simulink model "attitude_controllerV6"  (R2025a)
settings: Solver=FixedStepDiscrete  StartTime=0.0  StopTime=40  FixedStep=1e-4  RelTol=1e-6
undefined symbols (not defined in the file or in its folder): DiscIntNeverNeededParam
libraries: simulink x18, cstblocks x14, slpidlib x6, aerolibutil x2, rllib x1
(part 1 of 2)
settings Model: Creator=Rewse  LastModifiedBy=Rewse
settings SolverCC: ZeroCrossAlgorithm=Adaptive
settings DebuggingCC: IgnoredZcDiagnostic=none

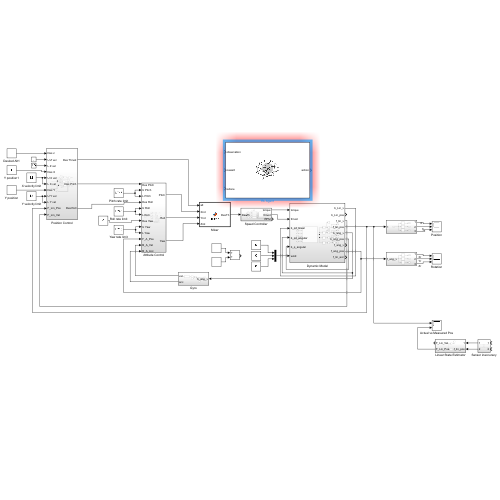
[thumbnail: Simulink's stored preview of the top-level diagram]
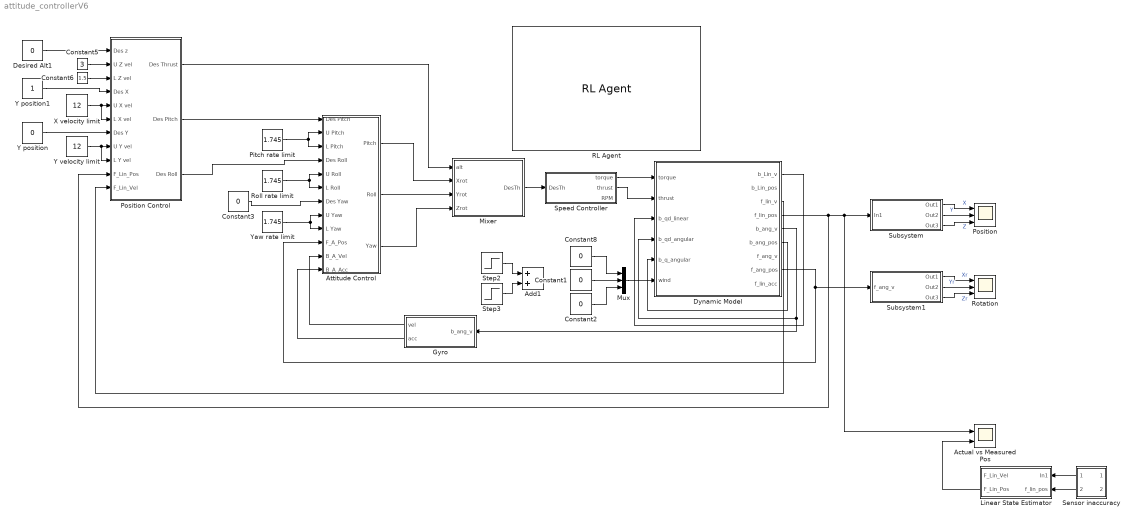
== system attitude_controllerV6 ==
  Actual vs Measured Pos : Scope  NumInputPorts=2
      settings: ActiveDisplayYMinimum=-0.72419600366773873  ActiveDisplayYMaximum=1.3775619520636175  DataLoggingVariableName=ScopeData20
  Add1 : Sum
  Attitude Control : Subsystem
  Constant{1..3,8} (4 alike) : Constant  Value=0
  Constant5 : Constant  Value=3
  Constant6 : Constant  Value=1.5
  Desired Alt1 : Constant  Value=0
  Dynamic Model : Subsystem
  Gyro : Subsystem
  Linear State Estimator : Subsystem
  Mixer : MATLAB Function  TreatAsAtomicUnit=on
  Mux : Mux  Inputs=3
  Pitch rate limit : Constant  Value=1.745
  Position : Scope  NumInputPorts=3
      settings: ActiveDisplayYMinimum=-0.995943473561637  ActiveDisplayYMaximum=3.6382297992423651
  Position Control : Subsystem
  RL Agent : rllib/RL Agent  Agent=agentObj  ExternalActionAsInput=off  ProvideLastAction=off  ProvideCumRwd=off  TreatAsDirectFeedthrough=on  UseStrictObservationDataTypes=off
  Roll rate limit : Constant  Value=1.745
  Rotation : Scope  NumInputPorts=3
      settings: ActiveDisplayYMinimum=-0.95912404587525768  ActiveDisplayYMaximum=0.95521723280052528
  Sensor inaccuracy : Subsystem
  Speed Controller : Subsystem
  Step2 : Step  After=15  SampleTime=2
  Step3 : Step  Time=8  After=-15  SampleTime=3
  Subsystem : Subsystem
  Subsystem1 : Subsystem
  X velocity limit : Constant  Value=12
  Y position : Constant  Value=0
  Y position1 : Constant
  Y velocity limit : Constant  Value=12
  Yaw rate limit : Constant  Value=1.745
  wires:
  Subsystem/1(Out1) -> Position/1  "X"
  Subsystem/2(Out2) -> Position/2  "Y"
  Subsystem/3(Out3) -> Position/3  "Z"
  Subsystem1/1(Out1) -> Rotation/1  "Xr"
  Subsystem1/2(Out2) -> Rotation/2  "Yr"
  Subsystem1/3(Out3) -> Rotation/3  "Zr"
  Dynamic Model/6(b_ang_pos) -> Dynamic Model/5(b_q_angular)
  Dynamic Model/1(b_Lin_v) -> Dynamic Model/3(b_qd_linear)
  Mixer/1(DesTh) -> Speed Controller/1(DesTh)
  Dynamic Model/5(b_ang_v) -> Dynamic Model/4(b_qd_angular), Gyro/1(b_ang_v)
  Attitude Control/1(Pitch) -> Mixer/2(Xrot)
  Attitude Control/2(Roll) -> Mixer/3(Yrot)
  Pitch rate limit/1 -> Attitude Control/3(L Pitch), Attitude Control/2(U Pitch)
  Roll rate limit/1 -> Attitude Control/6(L Roll), Attitude Control/5(U Roll)
  Yaw rate limit/1 -> Attitude Control/9(L Yaw), Attitude Control/8(U Yaw)
  Constant3/1 -> Attitude Control/7(Des Yaw)
  Mux/1 -> Dynamic Model/6(wind)
  Speed Controller/2(thrust) -> Dynamic Model/2(thrust)
  Speed Controller/1(torque) -> Dynamic Model/1(torque)
  Constant5/1 -> Position Control/2(U Z vel)
  Desired Alt1/1 -> Position Control/1(Des z)
  X velocity limit/1 -> Position Control/6(L X vel), Position Control/5(U X vel)
  Y velocity limit/1 -> Position Control/9(L Y vel), Position Control/8(U Y vel)
  Position Control/1(Des Thrust) -> Mixer/1(alt)
  Constant6/1 -> Position Control/3(L Z vel)
  Y position/1 -> Position Control/7(Des Y)
  Attitude Control/3(Yaw) -> Mixer/4(Zrot)
  Gyro/1(vel) -> Attitude Control/11(B_A_Vel)
  Gyro/2(acc) -> Attitude Control/12(B_A_Acc)
  Dynamic Model/8(f_ang_pos) -> Attitude Control/10(F_A_Pos), Subsystem1/1(f_ang_v)
  Y position1/1 -> Position Control/4(Des X)
  Constant2/1 -> Mux/3
  Constant8/1 -> Mux/1
  Step2/1 -> Add1/1
  Step3/1 -> Add1/2
  Sensor inaccuracy/2(Out2) -> Linear State Estimator/2(f_lin_pos)
  Sensor inaccuracy/1(Out1) -> Linear State Estimator/1(In1)
  Dynamic Model/3(f_lin_v) -> Position Control/11(F_Lin_Vel)
  Constant1/1 -> Mux/2
  Linear State Estimator/2(F_Lin_Pos) -> Actual vs Measured Pos/2
  Position Control/3(Des Roll) -> Attitude Control/4(Des Roll)
  Position Control/2(Des Pitch) -> Attitude Control/1(Des Pitch)
  Dynamic Model/4(f_lin_pos) -> Position Control/10(F_Lin_Pos), Actual vs Measured Pos/1, Subsystem/1(In1)

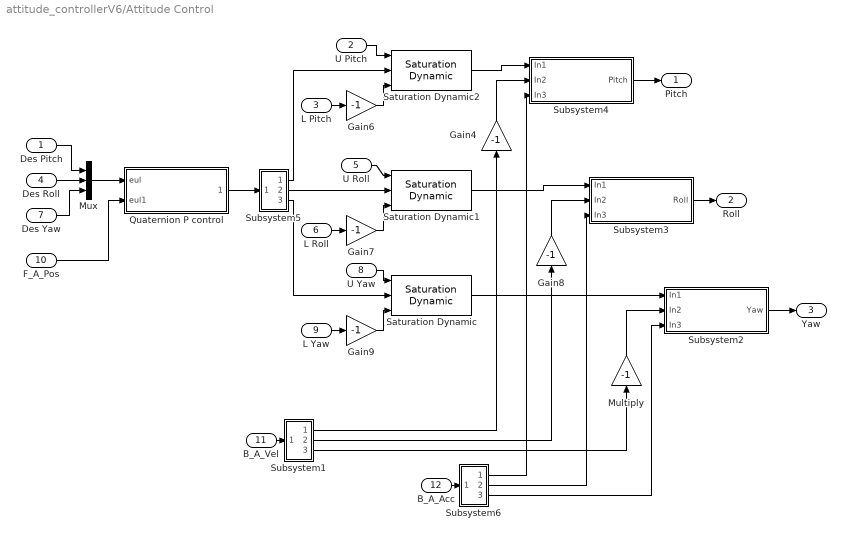
== system attitude_controllerV6/Attitude Control ==
  Des Pitch : Inport
  U Pitch : Inport  Port=2
  L Pitch : Inport  Port=3
  Des Roll : Inport  Port=4
  U Roll : Inport  Port=5
  L Roll : Inport  Port=6
  Des Yaw : Inport  Port=7
  U Yaw : Inport  Port=8
  L Yaw : Inport  Port=9
  F_A_Pos : Inport  Port=10
  B_A_Vel : Inport  Port=11
  B_A_Acc : Inport  Port=12
  Gain{4,6..9} (5 alike) : Gain  Gain=-1
  Multiply : Gain  Gain=-1
  Mux : Mux  Inputs=3
  Quaternion P control : Subsystem
  Saturation Dynamic : simulink/Discontinuities/Saturation Dynamic  OutMin=[]  OutMax=[]  OutDataTypeStr=Inherit: Same as second input  OutDataType=fixdt(1, 16)  OutScaling=2^-10  DoSatur=off
  Saturation Dynamic1 : simulink/Discontinuities/Saturation Dynamic  OutMin=[]  OutMax=[]  OutDataTypeStr=Inherit: Same as second input  OutDataType=fixdt(1, 16)  OutScaling=2^-10  DoSatur=off
  Saturation Dynamic2 : simulink/Discontinuities/Saturation Dynamic  OutMin=[]  OutMax=[]  OutDataTypeStr=Inherit: Same as second input  OutDataType=fixdt(1, 16)  OutScaling=2^-10  DoSatur=off
  Subsystem1 : Subsystem
  Subsystem2 : Subsystem
  Subsystem3 : Subsystem
  Subsystem4 : Subsystem
  Subsystem5 : Subsystem
  Subsystem6 : Subsystem
  Pitch : Outport
  Roll : Outport  Port=2
  Yaw : Outport  Port=3
  wires:
  Gain9/1 -> Saturation Dynamic/3
  Gain6/1 -> Saturation Dynamic2/3
  Gain7/1 -> Saturation Dynamic1/3
  B_A_Vel/1 -> Subsystem1/1("  ")
  U Roll/1 -> Saturation Dynamic1/1
  L Pitch/1 -> Gain6/1
  U Pitch/1 -> Saturation Dynamic2/1
  Subsystem1/1(Out1) -> Gain4/1
  Subsystem1/2(Out2) -> Gain8/1
  Subsystem1/3(Out3) -> Multiply/1
  Saturation Dynamic/1 -> Subsystem2/1(In1)
  Gain8/1 -> Subsystem3/2(In2)
  Subsystem2/1(Yaw) -> Yaw/1
  Multiply/1 -> Subsystem2/2(In2)
  Gain4/1 -> Subsystem4/2(In2)
  Subsystem4/1(Pitch) -> Pitch/1
  Saturation Dynamic1/1 -> Subsystem3/1(In1)
  Subsystem3/1(Roll) -> Roll/1
  L Yaw/1 -> Gain9/1
  Des Pitch/1 -> Mux/1
  Des Roll/1 -> Mux/2
  Des Yaw/1 -> Mux/3
  U Yaw/1 -> Saturation Dynamic/1
  Subsystem5/3(Out3) -> Saturation Dynamic/2
  Subsystem5/2(Out2) -> Saturation Dynamic1/2
  Subsystem5/1(Out1) -> Saturation Dynamic2/2
  Mux/1 -> Quaternion P control/1(eul)
  F_A_Pos/1 -> Quaternion P control/2(eul1)
  Quaternion P control/1("  ") -> Subsystem5/1("  ")
  L Roll/1 -> Gain7/1
  Saturation Dynamic2/1 -> Subsystem4/1(In1)
  B_A_Acc/1 -> Subsystem6/1("  ")
  Subsystem6/1(Out1) -> Subsystem4/3(In3)
  Subsystem6/2(Out2) -> Subsystem3/3(In3)
  Subsystem6/3(Out3) -> Subsystem2/3(In3)

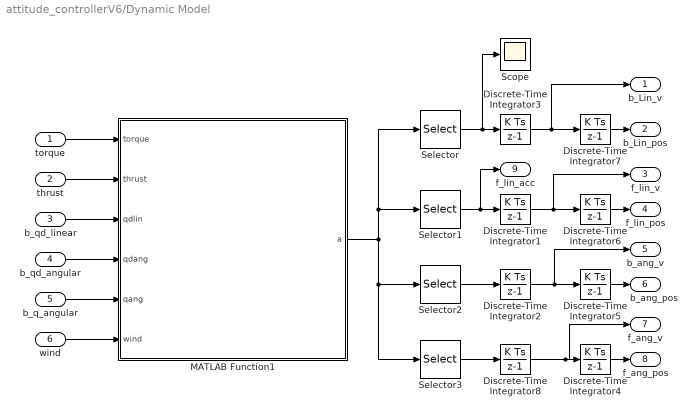
== system attitude_controllerV6/Dynamic Model ==
  torque : Inport
  thrust : Inport  Port=2
  b_qd_linear : Inport  Port=3
  b_qd_angular : Inport  Port=4
  b_q_angular : Inport  Port=5
  wind : Inport  Port=6
  Discrete-Time Integrator{1..8} (8 alike) : DiscreteIntegrator  SampleTime=-1  ICPrevOutput=DiscIntNeverNeededParam  ICPrevScaledInput=DiscIntNeverNeededParam
  MATLAB Function1 : MATLAB Function  TreatAsAtomicUnit=on
  Scope : Scope
      settings: ActiveDisplayYMinimum=-1  ActiveDisplayYMaximum=1  DataLoggingVariableName=ScopeData3
  Selector : Selector  InputPortWidth=12  IndexOptions=Index vector (dialog)  Indices=[1 2 3]  OutputSizes=1
  Selector1 : Selector  InputPortWidth=12  IndexOptions=Index vector (dialog)  Indices=[4 5 6]  OutputSizes=1
  Selector2 : Selector  InputPortWidth=12  IndexOptions=Index vector (dialog)  Indices=[7 8 9]  OutputSizes=1
  Selector3 : Selector  InputPortWidth=12  IndexOptions=Index vector (dialog)  Indices=[10 11 12]  OutputSizes=1
  b_Lin_v : Outport
  b_Lin_pos : Outport  Port=2
  f_lin_v : Outport  Port=3
  f_lin_pos : Outport  Port=4
  b_ang_v : Outport  Port=5
  b_ang_pos : Outport  Port=6
  f_ang_v : Outport  Port=7
  f_ang_pos : Outport  Port=8
  f_lin_acc : Outport  Port=9
  wires:
  torque/1 -> MATLAB Function1/1(torque)
  thrust/1 -> MATLAB Function1/2(thrust)
  b_qd_linear/1 -> MATLAB Function1/3(qdlin)
  b_qd_angular/1 -> MATLAB Function1/4(qdang)
  b_q_angular/1 -> MATLAB Function1/5(qang)
  wind/1 -> MATLAB Function1/6(wind)
  MATLAB Function1/1(a) -> Selector1/1, Selector/1, Selector3/1, Selector2/1
  Selector/1 -> Scope/1, Discrete-Time Integrator3/1
  Selector1/1 -> f_lin_acc/1, Discrete-Time Integrator1/1
  Selector2/1 -> Discrete-Time Integrator2/1
  Selector3/1 -> Discrete-Time Integrator8/1
  Discrete-Time Integrator3/1 -> Discrete-Time Integrator7/1, b_Lin_v/1
  Discrete-Time Integrator7/1 -> b_Lin_pos/1
  Discrete-Time Integrator2/1 -> b_ang_v/1, Discrete-Time Integrator5/1
  Discrete-Time Integrator1/1 -> Discrete-Time Integrator6/1, f_lin_v/1
  Discrete-Time Integrator8/1 -> f_ang_v/1, Discrete-Time Integrator4/1
  Discrete-Time Integrator4/1 -> f_ang_pos/1
  Discrete-Time Integrator5/1 -> b_ang_pos/1
  Discrete-Time Integrator6/1 -> f_lin_pos/1

== system attitude_controllerV6/Gyro ==
  b_ang_v : Inport
  Constant1 : Constant  Value=40
  Constant7 : Constant  Value=40
  Discrete Derivative : simulink/Discrete/Discrete Derivative  gainval=1.0  ICPrevScaledInput=0.0  OutMin=[]  OutMax=[]  OutDataType=fixdt(1, 16)  OutScaling=2^-10  DoSatur=off
  Discrete Varying Lowpass : cstblocks/Linear Parameter Varying/Discrete Varying Lowpass  N=2  w0=0  Ts=1e-3
  Discrete Varying Lowpass1 : cstblocks/Linear Parameter Varying/Discrete Varying Lowpass  N=2  w0=0  Ts=1e-3
  Quantizer : Quantizer  QuantizationInterval=0.00026179939
  noise : Subsystem
  vel : Outport
  acc : Outport  Port=2
  wires:
  Constant1/1 -> Discrete Varying Lowpass1/2
  Quantizer/1 -> Discrete Varying Lowpass/1
  Discrete Derivative/1 -> Discrete Varying Lowpass1/1
  Constant7/1 -> Discrete Varying Lowpass/2
  Discrete Varying Lowpass/1 -> vel/1, Discrete Derivative/1
  b_ang_v/1 -> noise/1(In1)
  noise/1(Out1) -> Quantizer/1
  Discrete Varying Lowpass1/1 -> acc/1

== system attitude_controllerV6/Linear State Estimator ==
  In1 : Inport
  f_lin_pos : Inport  Port=2
  Complimentary filter : Subsystem
  Constant7 : Constant  Value=10
  Discrete Varying Lowpass1 : cstblocks/Linear Parameter Varying/Discrete Varying Lowpass  N=2  w0=0  Ts=1e-3
  Scope : Scope
      settings: ActiveDisplayYMinimum=-0.34461683334154741  ActiveDisplayYMaximum=0.3611283671784512  DataLoggingVariableName=ScopeData17
  F_Lin_Vel : Outport
  F_Lin_Pos : Outport  Port=2
  wires:
  In1/1 -> Discrete Varying Lowpass1/1, Complimentary filter/1(In1)
  f_lin_pos/1 -> Complimentary filter/2(f_lin_pos)
  Complimentary filter/1(F_Lin_Pos) -> F_Lin_Pos/1
  Discrete Varying Lowpass1/1 -> Scope/1, F_Lin_Vel/1
  Constant7/1 -> Discrete Varying Lowpass1/2

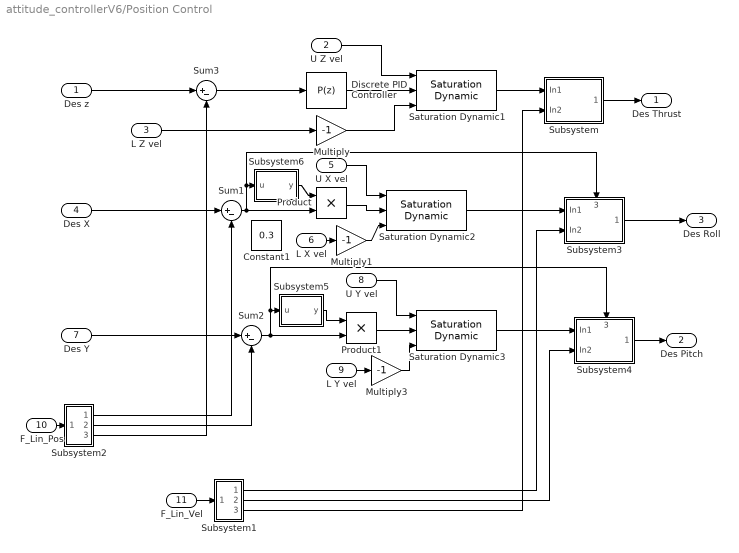
== system attitude_controllerV6/Position Control ==
  Des z : Inport
  U Z vel : Inport  Port=2
  L Z vel : Inport  Port=3
  Des X : Inport  Port=4
  U X vel : Inport  Port=5
  L X vel : Inport  Port=6
  Des Y : Inport  Port=7
  U Y vel : Inport  Port=8
  L Y vel : Inport  Port=9
  F_Lin_Pos : Inport  Port=10
  F_Lin_Vel : Inport  Port=11
  Constant1 : Constant  Value=0.3
  Discrete PID Controller : slpidlib/PID Controller  Controller=P  Form=Parallel  TimeDomain=Discrete-time  UseExternalTs=off  SampleTime=-1  IntegratorMethod=Forward Euler  FilterMethod=Forward Euler  ControllerParametersSource=internal  P=4  I=0.2  UseKiTs=off  D=1  UseExternalDerivativeSource=off  N=100  UseFilter=on  TunerSelectOption=Transfer Function Based (PID Tuner App)  InitialConditionSource=internal  InitialConditionForIntegrator=0  InitialConditionForFilter=0  DifferentiatorICPrevScaledInput=0  ExternalReset=none  TrackingMode=off  Kt=1  LimitOutput=off  SatLimitsSource=internal  UpperSaturationLimit=inf  LowerSaturationLimit=-inf  LinearizeAsGain=off  AntiWindupMode=none  Kb=1  LimitIntegrator=off  UpperIntegratorSaturationLimit=inf  LowerIntegratorSaturationLimit=-inf  POutMin=[]  POutMax=[]  IOutMin=[]  IOutMax=[]  DOutMin=[]  DOutMax=[]  NOutMin=[]  NOutMax=[]  SumOutMin=[]  SumOutMax=[]  SaturationOutMin=[]  SaturationOutMax=[]  PParamMin=[]  PParamMax=[]  IParamMin=[]  IParamMax=[]  DParamMin=[]  DParamMax=[]  NParamMin=[]  NParamMax=[]  KbParamMin=[]  KbParamMax=[]  KtParamMin=[]  KtParamMax=[]  KbOutMin=[]  KbOutMax=[]  KtOutMin=[]  KtOutMax=[]  IntegratorOutMin=[]  IntegratorOutMax=[]  FilterOutMin=[]  FilterOutMax=[]  SumI1OutMin=[]  SumI1OutMax=[]  SumI2OutMin=[]  SumI2OutMax=[]  SumI3OutMin=[]  SumI3OutMax=[]  SumI4OutMin=[]  SumI4OutMax=[]  SumDOutMin=[]  SumDOutMax=[]  DifferentiatorOutMin=[]  DifferentiatorOutMax=[]  FilterDiffOutCoefMin=[]  FilterDiffOutCoefMax=[]  ReciprocalOutMin=[]  ReciprocalOutMax=[]  SumDenOutMin=[]  SumDenOutMax=[]  SumNumOutMin=[]  SumNumOutMax=[]  DivideOutMin=[]  DivideOutMax=[]  UdiffTsProdOutMin=[]  UdiffTsProdOutMax=[]  NTsProdOutMin=[]  NTsProdOutMax=[]  UintegralTsProdOutMin=[]  UintegralTsProdOutMax=[]  UngainTsProdOutMin=[]  UngainTsProdOutMax=[]  ClampingZeroOutDataTypeStr=Inherit: Inherit via back propagation  ClampingZeroOutMin=[]  ClampingZeroOutMax=[]  FilterDenConstantOutDataTypeStr=Inherit: Inherit via back propagation  FilterDenConstantOutMin=[]  FilterDenConstantOutMax=[]  PCopyOutDataTypeStr=Inherit: Inherit via back propagation  PCopyOutMin=[]  PCopyOutMax=[]  NCopyOutDataTypeStr=Inherit: Inherit via back propagation  NCopyOutMin=[]  NCopyOutMax=[]  IntegratorContinuousStateAttributes=''  IntegratorStateMustResolveToSignalObject=off  IntegratorRTWStateStorageClass=Auto  FilterContinuousStateAttributes=''  FilterStateMustResolveToSignalObject=off  FilterRTWStateStorageClass=Auto  ParallelPVariant=InternalParameters  IdealPVariant=Disabled  IVariant=Disabled  DVariant=Disabled  IntegratorVariant=Disabled  SatVariant=Disabled  AWVariant=Disabled  PCopyVariant=Disabled  TRVariant=Disabled  FdbkBlocksVariant=Forward  IdealPFdbkVariant=Disabled  SatFdbkVariant=Disabled  DerivativeFilterVariant=Disabled  NVariant=Disabled  NCopyVariant=Disabled_SignalSpec  FilterICVariant=Disabled  IntegratorICVariant=Disabled  ExternalResetVariant=Disabled  TRSumVariant=Passthrough  SumFdbkVariant=Disabled  SumVariant=Passthrough_P  TsampFilterVariant=InternalTs  TsampNgainVariant=Passthrough  TsampIntegralVariant=Disabled_SignalSpec  ExternalSaturationOutDataTypeStr=Inherit: Same as second input  DerivativeSourceVariant=Disabled  PreIntVariant=InternalPreInt
      settings: LibrarySourceBlock=simulink/Discrete/Discrete PID Controller
  Multiply : Gain  Gain=-1
  Multiply1 : Gain  Gain=-1
  Multiply3 : Gain  Gain=-1
  Product : Product
  Product1 : Product
  Saturation Dynamic1 : simulink/Discontinuities/Saturation Dynamic  OutMin=[]  OutMax=[]  OutDataTypeStr=Inherit: Same as second input  OutDataType=fixdt(1, 16)  OutScaling=2^-10  DoSatur=off
  Saturation Dynamic2 : simulink/Discontinuities/Saturation Dynamic  OutMin=[]  OutMax=[]  OutDataTypeStr=Inherit: Same as second input  OutDataType=fixdt(1, 16)  OutScaling=2^-10  DoSatur=off
  Saturation Dynamic3 : simulink/Discontinuities/Saturation Dynamic  OutMin=[]  OutMax=[]  OutDataTypeStr=Inherit: Same as second input  OutDataType=fixdt(1, 16)  OutScaling=2^-10  DoSatur=off
  Subsystem : Subsystem
  Subsystem1 : Subsystem
  Subsystem2 : Subsystem
  Subsystem3 : Subsystem
      settings: PortSchema="{\"entries\":[{\"content\":{\"sides\":[{\"content\":{\"connectorIds\":[\"In1\",\"In2\"]},\"type\":\"ConnectorPlacement.EquallySpacedRectSide\",\"uuid\":\"8f94e582-882b-486f-b435-c6f08064346b\"},{\"content\":{\"connectorIds\":[\"Out1\"],\"side\":\"RIGHT\"},\"type\":\"ConnectorPlacement.EquallySpacedRectSide\",\"uuid\":\"472883df-7159-496e-9a5d-2a26c086a4a5\"},{\"content\":{\"connectorIds\":[\"In3\"],\"side\":\"TOP\"},\"type\":\"ConnectorPlacement.EquallySpacedRectSide\",\"uuid\":\"9ed532c8-9328-48c4-bd89-739726c76bc0\"}]},\"type\":\"ConnectorPlacement.EquallySpacedConnector\",\"uuid\":\"e990e484-f5ed-4898-afa7-038328da9bdf\"}],\"packageUris\":[\"http://schema.mathworks.com/mf0/Connector/R2020b\"],\"version\":\"1.0\"}"
  Subsystem4 : Subsystem
      settings: PortSchema="{\"entries\":[{\"content\":{\"sides\":[{\"content\":{\"connectorIds\":[\"In1\",\"In2\"]},\"type\":\"ConnectorPlacement.EquallySpacedRectSide\",\"uuid\":\"8f94e582-882b-486f-b435-c6f08064346b\"},{\"content\":{\"connectorIds\":[\"Out1\"],\"side\":\"RIGHT\"},\"type\":\"ConnectorPlacement.EquallySpacedRectSide\",\"uuid\":\"472883df-7159-496e-9a5d-2a26c086a4a5\"},{\"content\":{\"connectorIds\":[\"In3\"],\"side\":\"TOP\"},\"type\":\"ConnectorPlacement.EquallySpacedRectSide\",\"uuid\":\"9ed532c8-9328-48c4-bd89-739726c76bc0\"}]},\"type\":\"ConnectorPlacement.EquallySpacedConnector\",\"uuid\":\"e990e484-f5ed-4898-afa7-038328da9bdf\"}],\"packageUris\":[\"http://schema.mathworks.com/mf0/Connector/R2020b\"],\"version\":\"1.0\"}"
  Subsystem5 : Subsystem
  Subsystem6 : Subsystem
  Sum1 : Sum  Inputs=|+-
  Sum2 : Sum  Inputs=|+-
  Sum3 : Sum  Inputs=|+-
  Des Thrust : Outport
  Des Pitch : Outport  Port=2
  Des Roll : Outport  Port=3
  wires:
  Sum3/1 -> Discrete PID Controller/1
  Multiply/1 -> Saturation Dynamic1/3
  Des z/1 -> Sum3/1
  Discrete PID Controller/1 -> Saturation Dynamic1/2
  L Z vel/1 -> Multiply/1
  U Z vel/1 -> Saturation Dynamic1/1
  Saturation Dynamic1/1 -> Subsystem/1(In1)
  F_Lin_Vel/1 -> Subsystem1/1("  ")
  F_Lin_Pos/1 -> Subsystem2/1("  ")
  Subsystem2/3(Out3) -> Sum3/2
  Subsystem1/3(Out3) -> Subsystem/2(In2)
  Subsystem/1(Des Thrust) -> Des Thrust/1
  Des X/1 -> Sum1/1
  Sum1/1 -> Subsystem3/3(3), Subsystem6/1(u), Product/2
  Product/1 -> Saturation Dynamic2/2
  U X vel/1 -> Saturation Dynamic2/1
  Multiply1/1 -> Saturation Dynamic2/3
  L X vel/1 -> Multiply1/1
  Saturation Dynamic2/1 -> Subsystem3/1(In1)
  L Y vel/1 -> Multiply3/1
  Multiply3/1 -> Saturation Dynamic3/3
  Sum2/1 -> Subsystem5/1(u), Subsystem4/3(3), Product1/2
  Product1/1 -> Saturation Dynamic3/2
  Saturation Dynamic3/1 -> Subsystem4/1(In1)
  Subsystem4/1(Des Pitch) -> Des Pitch/1
  Des Y/1 -> Sum2/1
  U Y vel/1 -> Saturation Dynamic3/1
  Subsystem1/2(Out2) -> Subsystem4/2(In2)
  Subsystem1/1(Out1) -> Subsystem3/2(In2)
  Subsystem2/2(Out1) -> Sum2/2
  Subsystem2/1(Out2) -> Sum1/2
  Subsystem3/1(Des Roll) -> Des Roll/1
  Subsystem6/1(y) -> Product/1
  Subsystem5/1(y) -> Product1/1

== system attitude_controllerV6/Sensor inaccuracy ==
  In1 : Inport
  In2 : Inport  Port=2
  Quantizer : Quantizer  QuantizationInterval=0.01
  Quantizer1 : Quantizer  QuantizationInterval=1
  Out1 : Outport
  Out2 : Outport  Port=2
  wires:
  In1/1 -> Quantizer/1
  In2/1 -> Quantizer1/1
  Quantizer1/1 -> Out2/1
  Quantizer/1 -> Out1/1

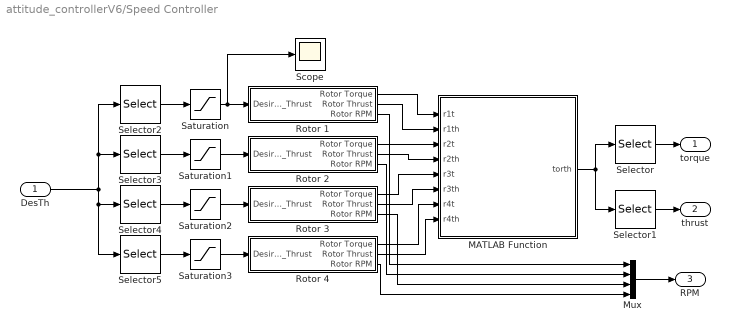
== system attitude_controllerV6/Speed Controller ==
  DesTh : Inport
  MATLAB Function : MATLAB Function  TreatAsAtomicUnit=on
  Mux : Mux
  Rotor 1 : Subsystem
  Rotor 2 : Subsystem
  Rotor 3 : Subsystem
  Rotor 4 : Subsystem
  Saturation{,1..3} (4 alike) : Saturate  UpperLimit=8.96325  LowerLimit=0
  Scope : Scope
      settings: ActiveDisplayYMinimum=-0.6431468749999999  ActiveDisplayYMaximum=5.788321875  DataLoggingVariableName=ScopeData6
  Selector : Selector  InputPortWidth=4  IndexOptions=Index vector (dialog)  Indices=[1 2 3]  OutputSizes=1
  Selector1 : Selector  InputPortWidth=4  IndexOptions=Index vector (dialog)  Indices=[4]  OutputSizes=1
  Selector2 : Selector  InputPortWidth=4  IndexOptions=Index vector (dialog)  Indices=[1]  OutputSizes=1
  Selector3 : Selector  InputPortWidth=4  IndexOptions=Index vector (dialog)  Indices=[2]  OutputSizes=1
  Selector4 : Selector  InputPortWidth=4  IndexOptions=Index vector (dialog)  Indices=[3]  OutputSizes=1
  Selector5 : Selector  InputPortWidth=4  IndexOptions=Index vector (dialog)  Indices=[4]  OutputSizes=1
  torque : Outport
  thrust : Outport  Port=2
  RPM : Outport  Port=3
  wires:
  DesTh/1 -> Selector5/1, Selector4/1, Selector3/1, Selector2/1
  Selector5/1 -> Saturation3/1
  Rotor 1/1(Rotor Torque) -> MATLAB Function/1(r1t)
  Selector2/1 -> Saturation/1
  Rotor 3/1(Rotor Torque) -> MATLAB Function/5(r3t)
  Selector3/1 -> Saturation1/1
  Rotor 1/2(Rotor Thrust) -> MATLAB Function/2(r1th)
  Selector4/1 -> Saturation2/1
  Rotor 2/1(Rotor Torque) -> MATLAB Function/3(r2t)
  MATLAB Function/1(torth) -> Selector/1, Selector1/1
  Selector1/1 -> thrust/1
  Selector/1 -> torque/1
  Saturation/1 -> Scope/1, Rotor 1/1(Desired_Thrust)
  Saturation1/1 -> Rotor 2/1(Desired_Thrust)
  Saturation2/1 -> Rotor 3/1(Desired_Thrust)
  Saturation3/1 -> Rotor 4/1(Desired_Thrust)
  Rotor 2/2(Rotor Thrust) -> MATLAB Function/4(r2th)
  Rotor 3/2(Rotor Thrust) -> MATLAB Function/6(r3th)
  Rotor 4/1(Rotor Torque) -> MATLAB Function/7(r4t)
  Rotor 4/2(Rotor Thrust) -> MATLAB Function/8(r4th)
  Rotor 1/3(Rotor RPM) -> Mux/1
  Rotor 2/3(Rotor RPM) -> Mux/2
  Rotor 3/3(Rotor RPM) -> Mux/3
  Rotor 4/3(Rotor RPM) -> Mux/4
  Mux/1 -> RPM/1

== system attitude_controllerV6/Subsystem ==
  In1 : Inport
  Selector1 : Selector  InputPortWidth=3  IndexOptions=Index vector (dialog)  Indices=[2]  OutputSizes=1
  Selector10 : Selector  InputPortWidth=3  IndexOptions=Index vector (dialog)  Indices=[1]  OutputSizes=1
  Selector2 : Selector  InputPortWidth=3  IndexOptions=Index vector (dialog)  Indices=[3]  OutputSizes=1
  Out1 : Outport
  Out2 : Outport  Port=2
  Out3 : Outport  Port=3
  wires:
  Selector10/1 -> Out1/1  "Xpos"
  Selector1/1 -> Out2/1  "Ypos"
  In1/1 -> Selector2/1, Selector10/1, Selector1/1
  Selector2/1 -> Out3/1  "Zpos"

== system attitude_controllerV6/Subsystem1 ==
  f_ang_v : Inport
  Selector1 : Selector  InputPortWidth=3  IndexOptions=Index vector (dialog)  Indices=[2]  OutputSizes=1
  Selector10 : Selector  InputPortWidth=3  IndexOptions=Index vector (dialog)  Indices=[1]  OutputSizes=1
  Selector2 : Selector  InputPortWidth=3  IndexOptions=Index vector (dialog)  Indices=[3]  OutputSizes=1
  Out1 : Outport
  Out2 : Outport  Port=2
  Out3 : Outport  Port=3
  wires:
  Selector10/1 -> Out1/1  "Xpos"
  Selector1/1 -> Out2/1  "Ypos"
  f_ang_v/1 -> Selector2/1, Selector10/1, Selector1/1
  Selector2/1 -> Out3/1  "Zpos"

== system attitude_controllerV6/Attitude Control/Quaternion P control ==
  eul : Inport
  eul1 : Inport  Port=2
  Discrete PID Controller1 : slpidlib/PID Controller  Controller=P  Form=Parallel  TimeDomain=Discrete-time  UseExternalTs=off  SampleTime=-1  IntegratorMethod=Forward Euler  FilterMethod=Forward Euler  ControllerParametersSource=internal  P=2  I=1  UseKiTs=off  D=0  UseExternalDerivativeSource=off  N=100  UseFilter=on  TunerSelectOption=Transfer Function Based (PID Tuner App)  InitialConditionSource=internal  InitialConditionForIntegrator=0  InitialConditionForFilter=0  DifferentiatorICPrevScaledInput=0  ExternalReset=none  TrackingMode=off  Kt=1  LimitOutput=off  SatLimitsSource=internal  UpperSaturationLimit=inf  LowerSaturationLimit=-inf  LinearizeAsGain=off  AntiWindupMode=none  Kb=1  LimitIntegrator=off  UpperIntegratorSaturationLimit=inf  LowerIntegratorSaturationLimit=-inf  POutMin=[]  POutMax=[]  IOutMin=[]  IOutMax=[]  DOutMin=[]  DOutMax=[]  NOutMin=[]  NOutMax=[]  SumOutMin=[]  SumOutMax=[]  SaturationOutMin=[]  SaturationOutMax=[]  PParamMin=[]  PParamMax=[]  IParamMin=[]  IParamMax=[]  DParamMin=[]  DParamMax=[]  NParamMin=[]  NParamMax=[]  KbParamMin=[]  KbParamMax=[]  KtParamMin=[]  KtParamMax=[]  KbOutMin=[]  KbOutMax=[]  KtOutMin=[]  KtOutMax=[]  IntegratorOutMin=[]  IntegratorOutMax=[]  FilterOutMin=[]  FilterOutMax=[]  SumI1OutMin=[]  SumI1OutMax=[]  SumI2OutMin=[]  SumI2OutMax=[]  SumI3OutMin=[]  SumI3OutMax=[]  SumI4OutMin=[]  SumI4OutMax=[]  SumDOutMin=[]  SumDOutMax=[]  DifferentiatorOutMin=[]  DifferentiatorOutMax=[]  FilterDiffOutCoefMin=[]  FilterDiffOutCoefMax=[]  ReciprocalOutMin=[]  ReciprocalOutMax=[]  SumDenOutMin=[]  SumDenOutMax=[]  SumNumOutMin=[]  SumNumOutMax=[]  DivideOutMin=[]  DivideOutMax=[]  UdiffTsProdOutMin=[]  UdiffTsProdOutMax=[]  NTsProdOutMin=[]  NTsProdOutMax=[]  UintegralTsProdOutMin=[]  UintegralTsProdOutMax=[]  UngainTsProdOutMin=[]  UngainTsProdOutMax=[]  ClampingZeroOutDataTypeStr=Inherit: Inherit via back propagation  ClampingZeroOutMin=[]  ClampingZeroOutMax=[]  FilterDenConstantOutDataTypeStr=Inherit: Inherit via back propagation  FilterDenConstantOutMin=[]  FilterDenConstantOutMax=[]  PCopyOutDataTypeStr=Inherit: Inherit via back propagation  PCopyOutMin=[]  PCopyOutMax=[]  NCopyOutDataTypeStr=Inherit: Inherit via back propagation  NCopyOutMin=[]  NCopyOutMax=[]  IntegratorContinuousStateAttributes=''  IntegratorStateMustResolveToSignalObject=off  IntegratorRTWStateStorageClass=Auto  FilterContinuousStateAttributes=''  FilterStateMustResolveToSignalObject=off  FilterRTWStateStorageClass=Auto  ParallelPVariant=InternalParameters  IdealPVariant=Disabled  IVariant=Disabled  DVariant=Disabled  IntegratorVariant=Disabled  SatVariant=Disabled  AWVariant=Disabled  PCopyVariant=Disabled  TRVariant=Disabled  FdbkBlocksVariant=Forward  IdealPFdbkVariant=Disabled  SatFdbkVariant=Disabled  DerivativeFilterVariant=Disabled  NVariant=Disabled  NCopyVariant=Disabled_SignalSpec  FilterICVariant=Disabled  IntegratorICVariant=Disabled  ExternalResetVariant=Disabled  TRSumVariant=Passthrough  SumFdbkVariant=Disabled  SumVariant=Passthrough_P  TsampFilterVariant=InternalTs  TsampNgainVariant=Passthrough  TsampIntegralVariant=Disabled_SignalSpec  ExternalSaturationOutDataTypeStr=Inherit: Same as second input  DerivativeSourceVariant=Disabled  PreIntVariant=InternalPreInt
      settings: LibrarySourceBlock=simulink/Discrete/Discrete PID Controller
  Gain2 : Gain  Gain=-1
  MATLAB Function : MATLAB Function  TreatAsAtomicUnit=on
  MATLAB Function1 : MATLAB Function  TreatAsAtomicUnit=on
  Product : Product
  Quaternion Inverse : aerolibutil/Quaternion Inverse
  Quaternion Multiplication : aerolibutil/Quaternion Multiplication
  Selector : Selector  InputPortWidth=4  IndexOptions=Index vector (dialog)  Indices=[1]  OutputSizes=1
  Selector1 : Selector  InputPortWidth=4  IndexOptions=Index vector (dialog)  Indices=[2 3 4]  OutputSizes=1
  Sign : Signum
  "  " : Outport
  wires:
  Quaternion Inverse/1 -> Quaternion Multiplication/2
  Selector1/1 -> Product/2
  Product/1 -> Discrete PID Controller1/1
  MATLAB Function/1(quat) -> Quaternion Multiplication/1
  MATLAB Function1/1(quat) -> Quaternion Inverse/1
  Quaternion Multiplication/1 -> Selector1/1, Selector/1
  Selector/1 -> Sign/1
  Discrete PID Controller1/1 -> Gain2/1
  Sign/1 -> Product/1
  Gain2/1 -> "  "/1
  eul/1 -> MATLAB Function/1(eul)
  eul1/1 -> MATLAB Function1/1(eul)

== system attitude_controllerV6/Attitude Control/Subsystem1 ==
  "  " : Inport
  Selector : Selector  InputPortWidth=3  IndexOptions=Index vector (dialog)  Indices=[1]  OutputSizes=1
  Selector1 : Selector  InputPortWidth=3  IndexOptions=Index vector (dialog)  Indices=[2]  OutputSizes=1
  Selector2 : Selector  InputPortWidth=3  IndexOptions=Index vector (dialog)  Indices=[3]  OutputSizes=1
  Out1 : Outport
  Out2 : Outport  Port=2
  Out3 : Outport  Port=3
  wires:
  Selector2/1 -> Out3/1
  Selector1/1 -> Out2/1
  Selector/1 -> Out1/1
  "  "/1 -> Selector2/1, Selector/1, Selector1/1

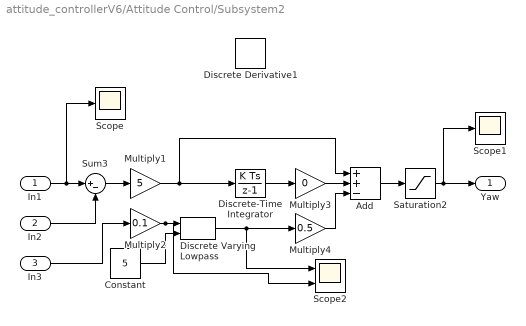
== system attitude_controllerV6/Attitude Control/Subsystem2 ==
  In1 : Inport
  In2 : Inport  Port=2
  In3 : Inport  Port=3
  Add : Sum  Inputs=++-
  Constant : Constant  Value=5
  Discrete Derivative1 : simulink/Discrete/Discrete Derivative  gainval=1.0  ICPrevScaledInput=0.0  OutMin=[]  OutMax=[]  OutDataType=fixdt(1, 16)  OutScaling=2^-10  DoSatur=off
  Discrete Varying Lowpass : cstblocks/Linear Parameter Varying/Discrete Varying Lowpass  N=1  w0=0  Ts=0.001
  Discrete-Time Integrator : DiscreteIntegrator  SampleTime=-1  ICPrevOutput=DiscIntNeverNeededParam  ICPrevScaledInput=DiscIntNeverNeededParam
  Multiply1 : Gain  Gain=5
  Multiply2 : Gain  Gain=0.1
  Multiply3 : Gain  Gain=0
  Multiply4 : Gain  Gain=0.5
  Saturation2 : Saturate  UpperLimit=20  LowerLimit=-20
  Scope : Scope
      settings: ActiveDisplayYMinimum=-0.62499999999786793  ActiveDisplayYMaximum=0.62499999998861677  DataLoggingVariableName=ScopeData8
  Scope1 : Scope
      settings: ActiveDisplayYMinimum=-1  ActiveDisplayYMaximum=1  DataLoggingVariableName=ScopeData9
  Scope2 : Scope  NumInputPorts=2
      settings: ActiveDisplayYMinimum=-1  ActiveDisplayYMaximum=1  DataLoggingVariableName=ScopeData19
  Sum3 : Sum  Inputs=|+-
  Yaw : Outport
  wires:
  In1/1 -> Scope/1, Sum3/1
  Sum3/1 -> Multiply1/1
  In2/1 -> Sum3/2
  Discrete-Time Integrator/1 -> Multiply3/1
  Multiply3/1 -> Add/2
  Discrete Varying Lowpass/1 -> Scope2/1, Multiply4/1
  Multiply1/1 -> Add/1, Discrete-Time Integrator/1
  Multiply4/1 -> Add/3
  Add/1 -> Saturation2/1
  Multiply2/1 -> Scope2/2, Discrete Varying Lowpass/1
  Constant/1 -> Discrete Varying Lowpass/2
  Saturation2/1 -> Scope1/1, Yaw/1
  In3/1 -> Multiply2/1

== system attitude_controllerV6/Attitude Control/Subsystem3 ==
  In1 : Inport
  In2 : Inport  Port=2
  In3 : Inport  Port=3
  Add : Sum  Inputs=++-
  Constant : Constant  Value=5
  Discrete Varying Lowpass : cstblocks/Linear Parameter Varying/Discrete Varying Lowpass  N=1  w0=0  Ts=0.001
  Discrete-Time Integrator : DiscreteIntegrator  SampleTime=-1  ICPrevOutput=DiscIntNeverNeededParam  ICPrevScaledInput=DiscIntNeverNeededParam
  Multiply1 : Gain  Gain=0.3
  Multiply2 : Gain  Gain=0.01
  Multiply3 : Gain  Gain=0
  Multiply4 : Gain
  Saturation2 : Saturate  UpperLimit=20  LowerLimit=-20
  Scope : Scope
      settings: ActiveDisplayYMinimum=-0.55681542497324932  ActiveDisplayYMaximum=0.063259639668785228  DataLoggingVariableName=ScopeData8
  Scope1 : Scope
      settings: ActiveDisplayYMinimum=-0.30519840806419729  ActiveDisplayYMaximum=0.27214507005405869  DataLoggingVariableName=ScopeData9
  Scope2 : Scope
      settings: ActiveDisplayYMinimum=-1  ActiveDisplayYMaximum=1  DataLoggingVariableName=ScopeData7
  Sum3 : Sum  Inputs=|+-
  Roll : Outport
  wires:
  In1/1 -> Scope/1, Sum3/1
  Sum3/1 -> Multiply1/1
  In2/1 -> Sum3/2
  Discrete-Time Integrator/1 -> Multiply3/1
  Multiply3/1 -> Add/2
  Discrete Varying Lowpass/1 -> Multiply4/1, Scope2/1
  Multiply1/1 -> Add/1, Discrete-Time Integrator/1
  Multiply4/1 -> Add/3
  Add/1 -> Saturation2/1
  Multiply2/1 -> Discrete Varying Lowpass/1
  Constant/1 -> Discrete Varying Lowpass/2
  Saturation2/1 -> Scope1/1, Roll/1
  In3/1 -> Multiply2/1

== system attitude_controllerV6/Attitude Control/Subsystem4 ==
  In1 : Inport
  In2 : Inport  Port=2
  In3 : Inport  Port=3
  Add : Sum  Inputs=++-
  Constant : Constant  Value=5
  Discrete Varying Lowpass : cstblocks/Linear Parameter Varying/Discrete Varying Lowpass  N=1  w0=0  Ts=0.001
  Discrete-Time Integrator : DiscreteIntegrator  SampleTime=-1  ICPrevOutput=DiscIntNeverNeededParam  ICPrevScaledInput=DiscIntNeverNeededParam
  Multiply1 : Gain  Gain=0.3
  Multiply2 : Gain  Gain=0.01
  Multiply3 : Gain  Gain=0
  Multiply4 : Gain
  Saturation2 : Saturate  UpperLimit=20  LowerLimit=-20
  Scope : Scope
      settings: ActiveDisplayYMinimum=-1  ActiveDisplayYMaximum=1  DataLoggingVariableName=ScopeData8
  Scope1 : Scope
      settings: ActiveDisplayYMinimum=-1.0247326439580651  ActiveDisplayYMaximum=0.497593795622584  DataLoggingVariableName=ScopeData9
  Scope2 : Scope  NumInputPorts=2
      settings: ActiveDisplayYMinimum=-1  ActiveDisplayYMaximum=1  DataLoggingVariableName=ScopeData18
  Sum3 : Sum  Inputs=|+-
  Pitch : Outport
  wires:
  In1/1 -> Scope/1, Sum3/1
  Sum3/1 -> Multiply1/1
  In2/1 -> Sum3/2
  Discrete-Time Integrator/1 -> Multiply3/1
  Multiply3/1 -> Add/2
  Discrete Varying Lowpass/1 -> Scope2/1, Multiply4/1
  Multiply1/1 -> Add/1, Discrete-Time Integrator/1
  Multiply4/1 -> Add/3
  Add/1 -> Saturation2/1
  Multiply2/1 -> Scope2/2, Discrete Varying Lowpass/1
  Constant/1 -> Discrete Varying Lowpass/2
  Saturation2/1 -> Scope1/1, Pitch/1
  In3/1 -> Multiply2/1

== system attitude_controllerV6/Attitude Control/Subsystem5 ==
  "  " : Inport
  Selector : Selector  InputPortWidth=3  IndexOptions=Index vector (dialog)  Indices=[1]  OutputSizes=1
  Selector1 : Selector  InputPortWidth=3  IndexOptions=Index vector (dialog)  Indices=[2]  OutputSizes=1
  Selector2 : Selector  InputPortWidth=3  IndexOptions=Index vector (dialog)  Indices=[3]  OutputSizes=1
  Out1 : Outport
  Out2 : Outport  Port=2
  Out3 : Outport  Port=3
  wires:
  Selector2/1 -> Out3/1
  Selector1/1 -> Out2/1
  Selector/1 -> Out1/1
  "  "/1 -> Selector2/1, Selector/1, Selector1/1

== system attitude_controllerV6/Attitude Control/Subsystem6 ==
  "  " : Inport
  Selector : Selector  InputPortWidth=3  IndexOptions=Index vector (dialog)  Indices=[1]  OutputSizes=1
  Selector1 : Selector  InputPortWidth=3  IndexOptions=Index vector (dialog)  Indices=[2]  OutputSizes=1
  Selector2 : Selector  InputPortWidth=3  IndexOptions=Index vector (dialog)  Indices=[3]  OutputSizes=1
  Out1 : Outport
  Out2 : Outport  Port=2
  Out3 : Outport  Port=3
  wires:
  "  "/1 -> Selector1/1, Selector/1, Selector2/1
  Selector/1 -> Out1/1
  Selector1/1 -> Out2/1
  Selector2/1 -> Out3/1

== system attitude_controllerV6/Gyro/noise ==
  In1 : Inport
  Add1 : Sum
  Add2 : Sum
  Add3 : Sum
  Band-Limited White Noise : simulink/Sources/Band-Limited White Noise  Cov=[1e-6]  Ts=1e-3  seed=[23341]
  Band-Limited White Noise1 : simulink/Sources/Band-Limited White Noise  Cov=[1e-6]  Ts=1e-3  seed=[23345]
  Band-Limited White Noise2 : simulink/Sources/Band-Limited White Noise  Cov=[1e-6]  Ts=1e-3  seed=[22341]
  Mux : Mux  Inputs=3
  Subsystem1 : Subsystem
  Out1 : Outport
  wires:
  In1/1 -> Subsystem1/1("  ")
  Mux/1 -> Out1/1
  Band-Limited White Noise/1 -> Add1/2
  Band-Limited White Noise1/1 -> Add2/2
  Band-Limited White Noise2/1 -> Add3/2
  Subsystem1/1(Out1) -> Add1/1
  Subsystem1/2(Out2) -> Add2/1
  Subsystem1/3(Out3) -> Add3/1
  Add1/1 -> Mux/1
  Add2/1 -> Mux/2
  Add3/1 -> Mux/3

== system attitude_controllerV6/Linear State Estimator/Complimentary filter ==
  In1 : Inport
  f_lin_pos : Inport  Port=2
  Constant : Constant  Value=2
  Discrete Transfer Fcn : DiscreteTransferFcn  Numerator=[4]  Denominator=[4 1]
  Discrete Varying Lowpass : cstblocks/Linear Parameter Varying/Discrete Varying Lowpass  N=1  w0=0  Ts=0.001
  Sum : Sum  Inputs=|++
  F_Lin_Pos : Outport
  wires:
  Constant/1 -> Discrete Varying Lowpass/2
  In1/1 -> Discrete Transfer Fcn/1
  Discrete Varying Lowpass/1 -> Sum/1
  Discrete Transfer Fcn/1 -> Sum/2
  f_lin_pos/1 -> Discrete Varying Lowpass/1
  Sum/1 -> F_Lin_Pos/1

== system attitude_controllerV6/Position Control/Subsystem ==
  In1 : Inport
  In2 : Inport  Port=2
  Add : Sum  Inputs=++-
  Constant : Constant  Value=5
  Discrete Derivative : simulink/Discrete/Discrete Derivative  gainval=1.0  ICPrevScaledInput=0.0  OutMin=[]  OutMax=[]  OutDataType=fixdt(1, 16)  OutScaling=2^-10  DoSatur=off
  Discrete Varying Lowpass : cstblocks/Linear Parameter Varying/Discrete Varying Lowpass  N=1  w0=0  Ts=1e-3
  Discrete-Time Integrator : DiscreteIntegrator  SampleTime=-1  ICPrevOutput=DiscIntNeverNeededParam  ICPrevScaledInput=DiscIntNeverNeededParam
  Multiply1 : Gain  Gain=0.15
  Multiply2 : Gain  Gain=0.3
  Multiply3 : Gain  Gain=12
  Scope : Scope
      settings: ActiveDisplayYMinimum=-3.139380998588098  ActiveDisplayYMaximum=28.25442898729289  DataLoggingVariableName=ScopeData10
  Scope1 : Scope
      settings: ActiveDisplayYMinimum=-0.53877163495337965  ActiveDisplayYMaximum=3.3931968483281532  DataLoggingVariableName=ScopeData11
  Sum : Sum  Inputs=|+-
  Des Thrust : Outport
  wires:
  In1/1 -> Scope1/1, Sum/1
  Discrete Varying Lowpass/1 -> Discrete Derivative/1
  Discrete Derivative/1 -> Multiply2/1
  Discrete-Time Integrator/1 -> Multiply1/1
  Sum/1 -> Multiply3/1
  Multiply3/1 -> Add/1, Discrete-Time Integrator/1
  Multiply1/1 -> Add/2
  Multiply2/1 -> Add/3
  Add/1 -> Scope/1, Des Thrust/1
  Constant/1 -> Discrete Varying Lowpass/2
  In2/1 -> Sum/2, Discrete Varying Lowpass/1

== system attitude_controllerV6/Position Control/Subsystem1 ==
  "  " : Inport
  Selector : Selector  InputPortWidth=3  IndexOptions=Index vector (dialog)  Indices=[1]  OutputSizes=1
  Selector1 : Selector  InputPortWidth=3  IndexOptions=Index vector (dialog)  Indices=[2]  OutputSizes=1
  Selector2 : Selector  InputPortWidth=3  IndexOptions=Index vector (dialog)  Indices=[3]  OutputSizes=1
  Out1 : Outport
  Out2 : Outport  Port=2
  Out3 : Outport  Port=3
  wires:
  Selector2/1 -> Out3/1
  Selector1/1 -> Out2/1
  Selector/1 -> Out1/1
  "  "/1 -> Selector2/1, Selector/1, Selector1/1

== system attitude_controllerV6/Position Control/Subsystem2 ==
  "  " : Inport
  Selector : Selector  InputPortWidth=3  IndexOptions=Index vector (dialog)  Indices=[1]  OutputSizes=1
  Selector1 : Selector  InputPortWidth=3  IndexOptions=Index vector (dialog)  Indices=[2]  OutputSizes=1
  Selector2 : Selector  InputPortWidth=3  IndexOptions=Index vector (dialog)  Indices=[3]  OutputSizes=1
  Out2 : Outport
  Out1 : Outport  Port=2
  Out3 : Outport  Port=3
  wires:
  Selector2/1 -> Out3/1
  "  "/1 -> Selector2/1, Selector/1, Selector1/1
  Selector1/1 -> Out1/1
  Selector/1 -> Out2/1

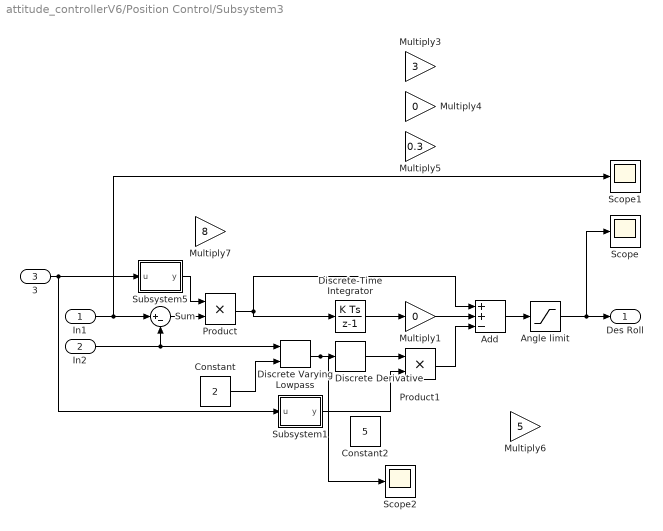
== system attitude_controllerV6/Position Control/Subsystem3 ==
  In1 : Inport
  In2 : Inport  Port=2
  3 : Inport  Port=3
  Add : Sum  Inputs=++-
  Angle limit : Saturate  UpperLimit=0.785  LowerLimit=-0.785
  Constant : Constant  Value=2
  Constant2 : Constant  Value=5
  Discrete Derivative : simulink/Discrete/Discrete Derivative  gainval=1.0  ICPrevScaledInput=0.0  OutMin=[]  OutMax=[]  OutDataType=fixdt(1, 16)  OutScaling=2^-10  DoSatur=off
  Discrete Varying Lowpass : cstblocks/Linear Parameter Varying/Discrete Varying Lowpass  N=1  w0=0  Ts=1e-3
  Discrete-Time Integrator : DiscreteIntegrator  SampleTime=-1  ICPrevOutput=DiscIntNeverNeededParam  ICPrevScaledInput=DiscIntNeverNeededParam
  Multiply1 : Gain  Gain=0
  Multiply3 : Gain  Gain=3
  Multiply4 : Gain  Gain=0
  Multiply5 : Gain  Gain=0.3
  Multiply6 : Gain  Gain=5
  Multiply7 : Gain  Gain=8
  Product : Product
  Product1 : Product
  Scope : Scope
      settings: ActiveDisplayYMinimum=-0.98125000000000007  ActiveDisplayYMaximum=0.98125000000000007  DataLoggingVariableName=ScopeData10
  Scope1 : Scope
      settings: ActiveDisplayYMinimum=-1  ActiveDisplayYMaximum=1  DataLoggingVariableName=ScopeData11
  Scope2 : Scope
      settings: ActiveDisplayYMinimum=-1  ActiveDisplayYMaximum=1  DataLoggingVariableName=ScopeData16
  Subsystem1 : Subsystem
  Subsystem5 : Subsystem
  Sum : Sum  Inputs=|+-
  Des Roll : Outport
  wires:
  Constant/1 -> Discrete Varying Lowpass/2
  Add/1 -> Angle limit/1
  Multiply1/1 -> Add/2
  Sum/1 -> Product/2
  Discrete-Time Integrator/1 -> Multiply1/1
  Discrete Derivative/1 -> Product1/1
  Discrete Varying Lowpass/1 -> Scope2/1, Discrete Derivative/1
  In1/1 -> Sum/1, Scope1/1
  Angle limit/1 -> Des Roll/1, Scope/1
  In2/1 -> Sum/2, Discrete Varying Lowpass/1
  Product/1 -> Discrete-Time Integrator/1, Add/1
  Subsystem5/1(y) -> Product/1
  Product1/1 -> Add/3
  Subsystem1/1(y) -> Product1/2
  3/1 -> Subsystem1/1(u), Subsystem5/1(u)

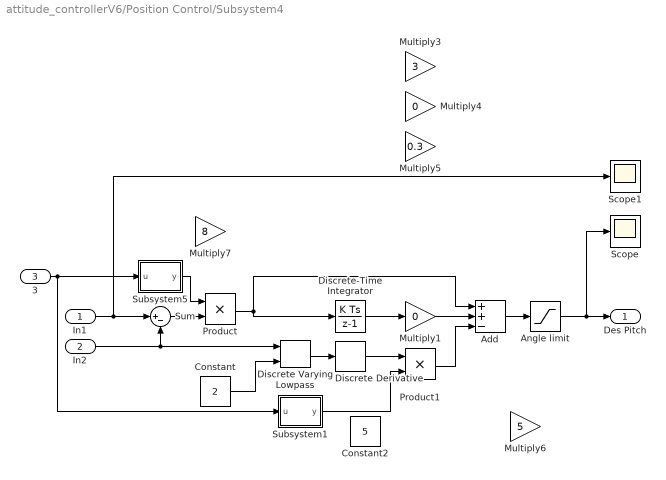
== system attitude_controllerV6/Position Control/Subsystem4 ==
  In1 : Inport
  In2 : Inport  Port=2
  3 : Inport  Port=3
  Add : Sum  Inputs=++-
  Angle limit : Saturate  UpperLimit=0.785  LowerLimit=-0.785
  Constant : Constant  Value=2
  Constant2 : Constant  Value=5
  Discrete Derivative : simulink/Discrete/Discrete Derivative  gainval=1.0  ICPrevScaledInput=0.0  OutMin=[]  OutMax=[]  OutDataType=fixdt(1, 16)  OutScaling=2^-10  DoSatur=off
  Discrete Varying Lowpass : cstblocks/Linear Parameter Varying/Discrete Varying Lowpass  N=1  w0=0  Ts=1e-3
  Discrete-Time Integrator : DiscreteIntegrator  SampleTime=-1  ICPrevOutput=DiscIntNeverNeededParam  ICPrevScaledInput=DiscIntNeverNeededParam
  Multiply1 : Gain  Gain=0
  Multiply3 : Gain  Gain=3
  Multiply4 : Gain  Gain=0
  Multiply5 : Gain  Gain=0.3
  Multiply6 : Gain  Gain=5
  Multiply7 : Gain  Gain=8
  Product : Product
  Product1 : Product
  Scope : Scope
      settings: ActiveDisplayYMinimum=-0.98125000000000007  ActiveDisplayYMaximum=0.98125000000000007  DataLoggingVariableName=ScopeData10
  Scope1 : Scope
      settings: ActiveDisplayYMinimum=-1  ActiveDisplayYMaximum=1  DataLoggingVariableName=ScopeData11
  Subsystem1 : Subsystem
  Subsystem5 : Subsystem
  Sum : Sum  Inputs=|+-
  Des Pitch : Outport
  wires:
  Subsystem1/1(y) -> Product1/2
  Product1/1 -> Add/3
  Subsystem5/1(y) -> Product/1
  3/1 -> Subsystem1/1(u), Subsystem5/1(u)
  Product/1 -> Add/1, Discrete-Time Integrator/1
  In2/1 -> Discrete Varying Lowpass/1, Sum/2
  Angle limit/1 -> Scope/1, Des Pitch/1
  In1/1 -> Scope1/1, Sum/1
  Discrete Varying Lowpass/1 -> Discrete Derivative/1
  Discrete Derivative/1 -> Product1/1
  Discrete-Time Integrator/1 -> Multiply1/1
  Sum/1 -> Product/2
  Multiply1/1 -> Add/2
  Add/1 -> Angle limit/1
  Constant/1 -> Discrete Varying Lowpass/2

== system attitude_controllerV6/Position Control/Subsystem5 ==
  u : Inport
  Abs1 : Abs  SaturateOnIntegerOverflow=off
  MATLAB Function : MATLAB Function  TreatAsAtomicUnit=on
  Scope : Scope
      settings: ActiveDisplayYMinimum=-1  ActiveDisplayYMaximum=1  DataLoggingVariableName=ScopeData2
  Scope1 : Scope
      settings: ActiveDisplayYMinimum=-1  ActiveDisplayYMaximum=1  DataLoggingVariableName=ScopeData14
  y : Outport
  wires:
  MATLAB Function/1(y) -> y/1, Scope/1
  u/1 -> Abs1/1
  Abs1/1 -> MATLAB Function/1(u), Scope1/1

== system attitude_controllerV6/Position Control/Subsystem6 ==
  u : Inport
  Abs1 : Abs  SaturateOnIntegerOverflow=off
  MATLAB Function : MATLAB Function  TreatAsAtomicUnit=on
  Scope : Scope
      settings: ActiveDisplayYMinimum=-1  ActiveDisplayYMaximum=1  DataLoggingVariableName=ScopeData2
  Scope1 : Scope
      settings: ActiveDisplayYMinimum=-1  ActiveDisplayYMaximum=1  DataLoggingVariableName=ScopeData14
  y : Outport
  wires:
  MATLAB Function/1(y) -> Scope/1, y/1
  u/1 -> Abs1/1
  Abs1/1 -> Scope1/1, MATLAB Function/1(u)

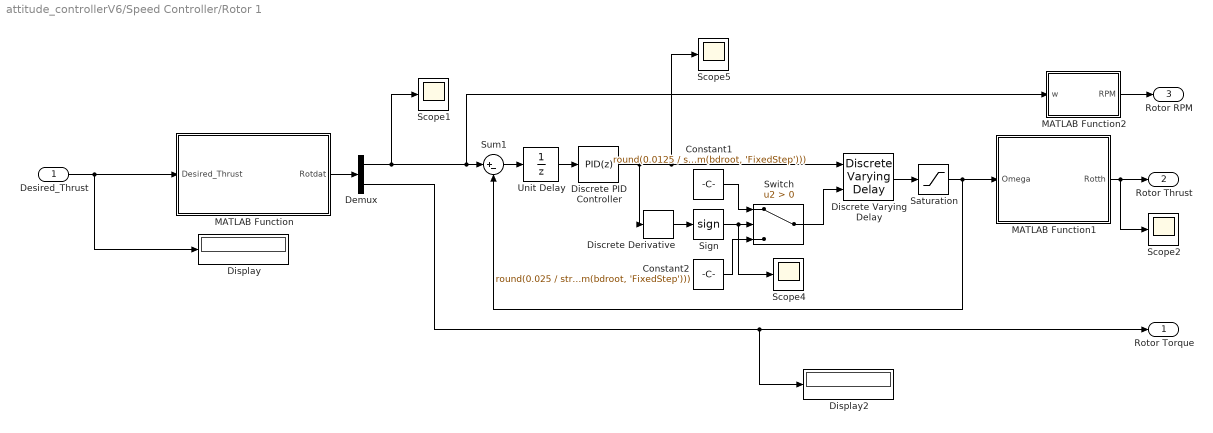
== system attitude_controllerV6/Speed Controller/Rotor 1 ==
  Desired_Thrust : Inport
  Constant1 : Constant  Value=round(0.0125 / str2double(get_param(bdroot, 'FixedStep')))
  Constant2 : Constant  Value=round(0.025 / str2double(get_param(bdroot, 'FixedStep')))
  Demux : Demux  Outputs=2
  Discrete Derivative : simulink/Discrete/Discrete Derivative  gainval=1.0  ICPrevScaledInput=0.0  OutMin=[]  OutMax=[]  OutDataType=fixdt(1, 16)  OutScaling=2^-10  DoSatur=off
  Discrete PID Controller : slpidlib/PID Controller  Controller=PID  Form=Parallel  TimeDomain=Discrete-time  UseExternalTs=off  SampleTime=-1  IntegratorMethod=Forward Euler  FilterMethod=Forward Euler  ControllerParametersSource=internal  P=0  I=30  UseKiTs=off  D=0  UseExternalDerivativeSource=off  N=100  UseFilter=on  TunerSelectOption=Transfer Function Based (PID Tuner App)  InitialConditionSource=internal  InitialConditionForIntegrator=0  InitialConditionForFilter=0  DifferentiatorICPrevScaledInput=0  ExternalReset=none  TrackingMode=off  Kt=1  LimitOutput=off  SatLimitsSource=internal  UpperSaturationLimit=inf  LowerSaturationLimit=-inf  LinearizeAsGain=off  AntiWindupMode=none  Kb=1  LimitIntegrator=off  UpperIntegratorSaturationLimit=inf  LowerIntegratorSaturationLimit=-inf  POutMin=[]  POutMax=[]  IOutMin=[]  IOutMax=[]  DOutMin=[]  DOutMax=[]  NOutMin=[]  NOutMax=[]  SumOutMin=[]  SumOutMax=[]  SaturationOutMin=[]  SaturationOutMax=[]  PParamMin=[]  PParamMax=[]  IParamMin=[]  IParamMax=[]  DParamMin=[]  DParamMax=[]  NParamMin=[]  NParamMax=[]  KbParamMin=[]  KbParamMax=[]  KtParamMin=[]  KtParamMax=[]  KbOutMin=[]  KbOutMax=[]  KtOutMin=[]  KtOutMax=[]  IntegratorOutMin=[]  IntegratorOutMax=[]  FilterOutMin=[]  FilterOutMax=[]  SumI1OutMin=[]  SumI1OutMax=[]  SumI2OutMin=[]  SumI2OutMax=[]  SumI3OutMin=[]  SumI3OutMax=[]  SumI4OutMin=[]  SumI4OutMax=[]  SumDOutMin=[]  SumDOutMax=[]  DifferentiatorOutMin=[]  DifferentiatorOutMax=[]  FilterDiffOutCoefMin=[]  FilterDiffOutCoefMax=[]  ReciprocalOutMin=[]  ReciprocalOutMax=[]  SumDenOutMin=[]  SumDenOutMax=[]  SumNumOutMin=[]  SumNumOutMax=[]  DivideOutMin=[]  DivideOutMax=[]  UdiffTsProdOutMin=[]  UdiffTsProdOutMax=[]  NTsProdOutMin=[]  NTsProdOutMax=[]  UintegralTsProdOutMin=[]  UintegralTsProdOutMax=[]  UngainTsProdOutMin=[]  UngainTsProdOutMax=[]  ClampingZeroOutDataTypeStr=Inherit: Inherit via back propagation  ClampingZeroOutMin=[]  ClampingZeroOutMax=[]  FilterDenConstantOutDataTypeStr=Inherit: Inherit via back propagation  FilterDenConstantOutMin=[]  FilterDenConstantOutMax=[]  PCopyOutDataTypeStr=Inherit: Inherit via back propagation  PCopyOutMin=[]  PCopyOutMax=[]  NCopyOutDataTypeStr=Inherit: Inherit via back propagation  NCopyOutMin=[]  NCopyOutMax=[]  IntegratorContinuousStateAttributes=''  IntegratorStateMustResolveToSignalObject=off  IntegratorRTWStateStorageClass=Auto  FilterContinuousStateAttributes=''  FilterStateMustResolveToSignalObject=off  FilterRTWStateStorageClass=Auto  ParallelPVariant=InternalParameters  IdealPVariant=Disabled  IVariant=InternalParameters  DVariant=InternalParameters  IntegratorVariant=Discrete  SatVariant=Disabled  AWVariant=Passthrough  PCopyVariant=Disabled  TRVariant=Disabled  FdbkBlocksVariant=Forward  IdealPFdbkVariant=Disabled  SatFdbkVariant=Disabled  DerivativeFilterVariant=ForwardEulerFilter  NVariant=InternalParameters  NCopyVariant=Disabled  FilterICVariant=InternalICsFilter  IntegratorICVariant=InternalICs  ExternalResetVariant=Disabled  TRSumVariant=Passthrough  SumFdbkVariant=Disabled  SumVariant=Sum_PID  TsampFilterVariant=InternalTs  TsampNgainVariant=Passthrough  TsampIntegralVariant=Disabled_SignalSpec  ExternalSaturationOutDataTypeStr=Inherit: Same as second input  DerivativeSourceVariant=ErrorSignal  PreIntVariant=InternalPreInt
      settings: LibrarySourceBlock=simulink/Discrete/Discrete PID Controller
  Discrete Varying Delay : cstblocks/Linear Parameter Varying/Discrete Varying Delay  Td=1  TdMax=10  TdFixed=[]  u0=0  Ts=-1  PreventDirectFeedthrough=off
  Display : Display
  Display2 : Display
  MATLAB Function : MATLAB Function  TreatAsAtomicUnit=on
  MATLAB Function1 : MATLAB Function  TreatAsAtomicUnit=on
  MATLAB Function2 : MATLAB Function  TreatAsAtomicUnit=on
  Saturation : Saturate  UpperLimit=1100  LowerLimit=0
  Scope{1..2,4..5} (4 alike) : Scope
      Scope1 settings: ActiveDisplayYMinimum=-154.8589621534594  ActiveDisplayYMaximum=1393.730659381135  DataLoggingVariableName=ScopeData4
      Scope2 settings: ActiveDisplayYMinimum=-0.6507136238694633  ActiveDisplayYMaximum=5.8564226148251706  DataLoggingVariableName=ScopeData5
      Scope4 settings: ActiveDisplayYMinimum=-1  ActiveDisplayYMaximum=1  DataLoggingVariableName=ScopeData12
      Scope5 settings: ActiveDisplayYMinimum=-115.66192536632313  ActiveDisplayYMaximum=1040.9573282969084  DataLoggingVariableName=ScopeData13
  Sign : Signum
  Sum1 : Sum  Inputs=|+-
  Switch : Switch  Criteria=u2 > Threshold  SaturateOnIntegerOverflow=off  InputSameDT=off
  Unit Delay : UnitDelay  SampleTime=-1  HasFrameUpgradeWarning=on
  Rotor Torque : Outport
  Rotor Thrust : Outport  Port=2
  Rotor RPM : Outport  Port=3
  wires:
  Demux/1 -> MATLAB Function2/1(w), Sum1/1, Scope1/1
  MATLAB Function1/1(Rotth) -> Rotor Thrust/1, Scope2/1
  MATLAB Function/1(Rotdat) -> Demux/1
  Desired_Thrust/1 -> Display/1, MATLAB Function/1(Desired_Thrust)
  Demux/2 -> Display2/1, Rotor Torque/1
  Saturation/1 -> MATLAB Function1/1(Omega), Sum1/2
  Sum1/1 -> Unit Delay/1
  Switch/1 -> Discrete Varying Delay/2
  Unit Delay/1 -> Discrete PID Controller/1
  Constant2/1 -> Switch/3
  Discrete Varying Delay/1 -> Saturation/1
  Discrete Derivative/1 -> Sign/1
  Constant1/1 -> Switch/1
  Discrete PID Controller/1 -> Scope5/1, Discrete Varying Delay/1, Discrete Derivative/1
  Sign/1 -> Scope4/1, Switch/2
  MATLAB Function2/1(RPM) -> Rotor RPM/1
